simulink model "simulink6"  (R2017b)
settings: Solver=VariableStepAuto  StartTime=0.0  StopTime=15  RelTol=1e-3
values from neighbouring files (symbols this model uses):
  P1 = [1 0 -p2 -p3]    [Uloha7.m]    (also in ulo.m = [1 0 -p1 -p2]; uloha6.m)
  P1New = [1 0 -p2New -p3New]    [uloha6.m]
  Q = [q0 q1 q2]    [Uloha7.m]    (also in ulo.m; uloha6.m)
  QNew = [q0New q1New q2New]    [uloha6.m]
settings Model: Creator=jan.sedivy  LastModifiedBy=jan.sedivy

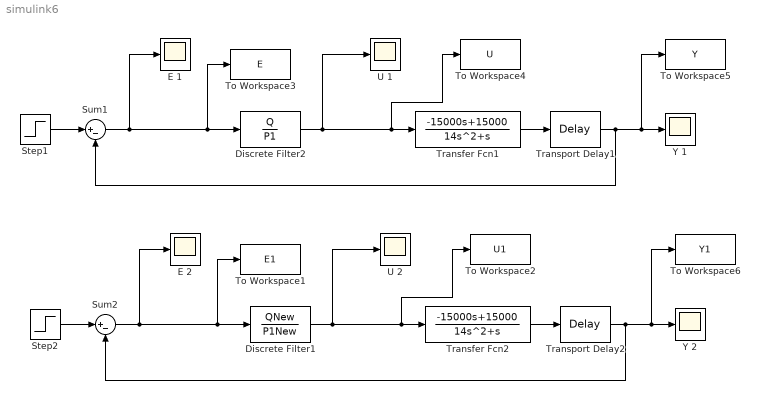
== system simulink6 ==
  Discrete Filter1 : DiscreteFilter  Numerator=QNew  Denominator=P1New  SampleTime=3
  Discrete Filter2 : DiscreteFilter  Numerator=Q  Denominator=P1  SampleTime=1
  E 1 : Scope
  E 2 : Scope
  Step1 : Step  Time=0  SampleTime=0
  Step2 : Step  Time=0  SampleTime=0
  Sum1 : Sum  Inputs=|+-
  Sum2 : Sum  Inputs=|+-
  To Workspace1 : ToWorkspace  VariableName=E1  SaveFormat=Timeseries  SampleTime=-1
  To Workspace2 : ToWorkspace  VariableName=U1  SaveFormat=Timeseries  SampleTime=-1
  To Workspace3 : ToWorkspace  VariableName=E  SaveFormat=Timeseries  SampleTime=-1
  To Workspace4 : ToWorkspace  VariableName=U  SaveFormat=Timeseries  SampleTime=-1
  To Workspace5 : ToWorkspace  VariableName=Y  SaveFormat=Timeseries  SampleTime=-1
  To Workspace6 : ToWorkspace  VariableName=Y1  SaveFormat=Timeseries  SampleTime=-1
  Transfer Fcn1 : TransferFcn  Numerator=[-15000 15000]  Denominator=[14 1 0]
  Transfer Fcn2 : TransferFcn  Numerator=[-15000 15000]  Denominator=[14 1 0]
  Transport Delay1 : TransportDelay
  Transport Delay2 : TransportDelay
  U 1 : Scope
  U 2 : Scope
  Y 1 : Scope
  Y 2 : Scope
  wires:
  Discrete Filter2/1 -> U 1/1, To Workspace4/1, Transfer Fcn1/1
  Transport Delay1/1 -> Sum1/2, To Workspace5/1, Y 1/1
  Step1/1 -> Sum1/1
  Transfer Fcn1/1 -> Transport Delay1/1
  Sum1/1 -> Discrete Filter2/1, To Workspace3/1, E 1/1
  Discrete Filter1/1 -> U 2/1, To Workspace2/1, Transfer Fcn2/1
  Transport Delay2/1 -> Sum2/2, To Workspace6/1, Y 2/1
  Step2/1 -> Sum2/1
  Transfer Fcn2/1 -> Transport Delay2/1
  Sum2/1 -> Discrete Filter1/1, To Workspace1/1, E 2/1
